simulink model "spring_network"  (R2021b)
settings: Solver=FixedStepAuto  StartTime=0.0  StopTime=10  FixedStep=5e-3  RelTol=1e-3
values from neighbouring files (symbols this model uses):
  dx0 = zeros(size(x_rest))    [gather_test_data.m]    (also in run_simulations.m = zeros(size(x0)); simulate_system.m = out.dx(end, :)')
  x0 = xs(start_step_idx, :)    [control_experiments.m]    (also in gather_test_data.m = x_rest; run_simulations.m; simulate_reduced.m = x0(1, :)'; simulate_system.m = out.x(end, :)')
undefined symbols (not defined in the file or in its folder): dynamics
settings Model: Creator=lepri  LastModifiedBy=lepri
settings DataIOCC: SaveOutput=off  SignalLogging=off  DSMLogging=off

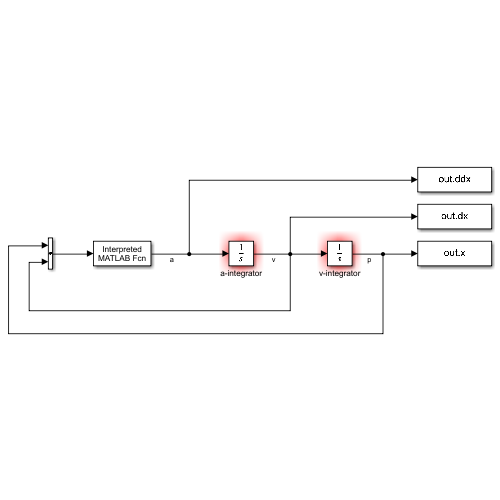
[thumbnail: Simulink's stored preview of the top-level diagram]
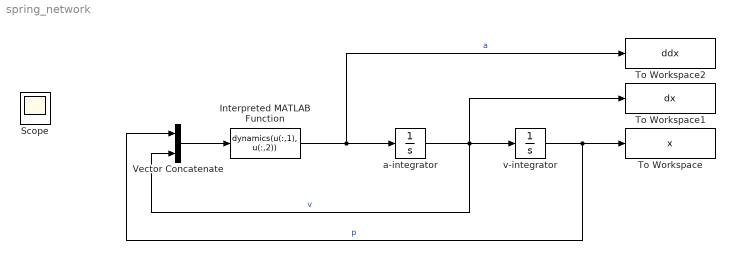
== system spring_network ==
  Interpreted MATLAB Function : MATLABFcn  MATLABFcn=dynamics(u(:,1), u(:,2))
  To Workspace : ToWorkspace  VariableName=x  SampleTime=-1
  To Workspace1 : ToWorkspace  VariableName=dx  SampleTime=-1
  To Workspace2 : ToWorkspace  VariableName=ddx  SampleTime=-1
  Vector Concatenate : Concatenate  Mode=Multidimensional array  ConcatenateDimension=2
  a-integrator : Integrator  InitialCondition=dx0  ContinuousStateAttributes='velocity'
  v-integrator : Integrator  InitialCondition=x0  ContinuousStateAttributes='position'
  Scope : Scope
  wires:
  a-integrator/1 -> To Workspace1/1, Vector Concatenate/2, v-integrator/1  "v"
  v-integrator/1 -> Vector Concatenate/1, To Workspace/1  "p"
  Interpreted MATLAB Function/1 -> To Workspace2/1, a-integrator/1  "a"
  Vector Concatenate/1 -> Interpreted MATLAB Function/1
